simulink model "TBS_SIM"  (R2016b)
settings: Solver=ode5  StartTime=15  StopTime=30  FixedStep=0.002  RelTol=1e-3
PreLoadFcn:
  | TBS_Cai_simu_init_20170316
InitFcn:
  | TBS_Cai_simu_init_20170214
StopFcn:
  | TBS_SIMULATION_LOG
undefined symbols (not defined in the file): air_density, L1X, L2X, L3X, L3Y, MAC1, MAC2, MAC3, magnitude, motor_m0, motor_t0, ORIGIN_CD, ORIGIN_CL, ORIGIN_CM, S_seg1, S_seg2, S_seg3, y_ac
libraries: aerolibconvert2 x20, simulink x13, aerolibtransform2 x4, aerolibwind2 x3, aerolib6dof2 x1, aerolibasang x1
(part 2 of 2)

== system TBS_SIM/Variant Control System/PIDcruise/Subsystem ==
  Euler : Inport
  Constant : Constant  Value=0
  Constant1 : Constant  Value=8
  Constant2 : Constant  Value=0
  Demux : Demux  Outputs=3
  Mux : Mux  Inputs=3
  PID Controller : simulink/Continuous/PID Controller  Controller=PID  TimeDomain=Continuous-time  SampleTime=-1  IntegratorMethod=Forward Euler  FilterMethod=Forward Euler  Form=Parallel  UseFilter=on  ControllerParametersSource=internal  P=0.5  I=0.1  D=0.01  N=100  InitialConditionSource=internal  InitialConditionForIntegrator=0  InitialConditionForFilter=0  ExternalReset=none  LimitOutput=off  UpperSaturationLimit=inf  LowerSaturationLimit=-inf  LinearizeAsGain=on  AntiWindupMode=none  Kb=1  TrackingMode=off  Kt=1  PParamMin=[]  PParamMax=[]  IParamMin=[]  IParamMax=[]  DParamMin=[]  DParamMax=[]  NParamMin=[]  NParamMax=[]  KbParamMin=[]  KbParamMax=[]  KtParamMin=[]  KtParamMax=[]  POutMin=[]  POutMax=[]  IOutMin=[]  IOutMax=[]  DOutMin=[]  DOutMax=[]  NOutMin=[]  NOutMax=[]  KbOutMin=[]  KbOutMax=[]  KtOutMin=[]  KtOutMax=[]  IntegratorOutMin=[]  IntegratorOutMax=[]  FilterOutMin=[]  FilterOutMax=[]  SumOutMin=[]  SumOutMax=[]  SumI1OutMin=[]  SumI1OutMax=[]  SumI2OutMin=[]  SumI2OutMax=[]  SumI3OutMin=[]  SumI3OutMax=[]  SumDOutMin=[]  SumDOutMax=[]  SaturationOutMin=[]  SaturationOutMax=[]  IntegratorContinuousStateAttributes=''  IntegratorStateMustResolveToSignalObject=off  IntegratorRTWStateStorageClass=Auto  FilterContinuousStateAttributes=''  FilterStateMustResolveToSignalObject=off  FilterRTWStateStorageClass=Auto  DifferentiatorICPrevScaledInput=0  DifferentiatorOutMin=[]  DifferentiatorOutMax=[]
  PID Controller1 : simulink/Continuous/PID Controller  Controller=PID  TimeDomain=Continuous-time  SampleTime=-1  IntegratorMethod=Forward Euler  FilterMethod=Forward Euler  Form=Parallel  UseFilter=on  ControllerParametersSource=internal  P=0.8  I=0.5  D=0.005  N=100  InitialConditionSource=internal  InitialConditionForIntegrator=0  InitialConditionForFilter=0  ExternalReset=none  LimitOutput=off  UpperSaturationLimit=inf  LowerSaturationLimit=-inf  LinearizeAsGain=on  AntiWindupMode=none  Kb=1  TrackingMode=off  Kt=1  PParamMin=[]  PParamMax=[]  IParamMin=[]  IParamMax=[]  DParamMin=[]  DParamMax=[]  NParamMin=[]  NParamMax=[]  KbParamMin=[]  KbParamMax=[]  KtParamMin=[]  KtParamMax=[]  POutMin=[]  POutMax=[]  IOutMin=[]  IOutMax=[]  DOutMin=[]  DOutMax=[]  NOutMin=[]  NOutMax=[]  KbOutMin=[]  KbOutMax=[]  KtOutMin=[]  KtOutMax=[]  IntegratorOutMin=[]  IntegratorOutMax=[]  FilterOutMin=[]  FilterOutMax=[]  SumOutMin=[]  SumOutMax=[]  SumI1OutMin=[]  SumI1OutMax=[]  SumI2OutMin=[]  SumI2OutMax=[]  SumI3OutMin=[]  SumI3OutMax=[]  SumDOutMin=[]  SumDOutMax=[]  SaturationOutMin=[]  SaturationOutMax=[]  IntegratorContinuousStateAttributes=''  IntegratorStateMustResolveToSignalObject=off  IntegratorRTWStateStorageClass=Auto  FilterContinuousStateAttributes=''  FilterStateMustResolveToSignalObject=off  FilterRTWStateStorageClass=Auto  DifferentiatorICPrevScaledInput=0  DifferentiatorOutMin=[]  DifferentiatorOutMax=[]
  PID Controller2 : simulink/Continuous/PID Controller  Controller=PID  TimeDomain=Continuous-time  SampleTime=-1  IntegratorMethod=Forward Euler  FilterMethod=Forward Euler  Form=Parallel  UseFilter=on  ControllerParametersSource=internal  P=3  I=1.5  D=0.5  N=100  InitialConditionSource=internal  InitialConditionForIntegrator=0  InitialConditionForFilter=0  ExternalReset=none  LimitOutput=off  UpperSaturationLimit=inf  LowerSaturationLimit=-inf  LinearizeAsGain=on  AntiWindupMode=none  Kb=1  TrackingMode=off  Kt=1  PParamMin=[]  PParamMax=[]  IParamMin=[]  IParamMax=[]  DParamMin=[]  DParamMax=[]  NParamMin=[]  NParamMax=[]  KbParamMin=[]  KbParamMax=[]  KtParamMin=[]  KtParamMax=[]  POutMin=[]  POutMax=[]  IOutMin=[]  IOutMax=[]  DOutMin=[]  DOutMax=[]  NOutMin=[]  NOutMax=[]  KbOutMin=[]  KbOutMax=[]  KtOutMin=[]  KtOutMax=[]  IntegratorOutMin=[]  IntegratorOutMax=[]  FilterOutMin=[]  FilterOutMax=[]  SumOutMin=[]  SumOutMax=[]  SumI1OutMin=[]  SumI1OutMax=[]  SumI2OutMin=[]  SumI2OutMax=[]  SumI3OutMin=[]  SumI3OutMax=[]  SumDOutMin=[]  SumDOutMax=[]  SaturationOutMin=[]  SaturationOutMax=[]  IntegratorContinuousStateAttributes=''  IntegratorStateMustResolveToSignalObject=off  IntegratorRTWStateStorageClass=Auto  FilterContinuousStateAttributes=''  FilterStateMustResolveToSignalObject=off  FilterRTWStateStorageClass=Auto  DifferentiatorICPrevScaledInput=0  DifferentiatorOutMin=[]  DifferentiatorOutMax=[]
  Sum : Sum  Inputs=+-|
  Sum1 : Sum  Inputs=+-|
  Sum2 : Sum  Inputs=+-|
  Out1 : Outport
  wires:
  Euler/1 -> Demux/1
  Sum/1 -> PID Controller/1
  Demux/1 -> Sum/2
  Constant/1 -> Sum/1
  Sum1/1 -> PID Controller1/1
  Demux/2 -> Sum1/2
  Constant1/1 -> Sum1/1
  Sum2/1 -> PID Controller2/1
  Demux/3 -> Sum2/2
  Constant2/1 -> Sum2/1
  PID Controller/1 -> Mux/1
  PID Controller1/1 -> Mux/2
  PID Controller2/1 -> Mux/3
  Mux/1 -> Out1/1

== system TBS_SIM/Variant Control System/PIDcruise/Subsystem1 ==
  Velocity : Inport
  Constant : Constant  Value=10
  PID Controller2 : simulink/Continuous/PID Controller  Controller=PID  TimeDomain=Continuous-time  SampleTime=-1  IntegratorMethod=Forward Euler  FilterMethod=Forward Euler  Form=Parallel  UseFilter=on  ControllerParametersSource=internal  P=3  I=1  D=0.5  N=100  InitialConditionSource=internal  InitialConditionForIntegrator=0  InitialConditionForFilter=0  ExternalReset=none  LimitOutput=off  UpperSaturationLimit=inf  LowerSaturationLimit=-inf  LinearizeAsGain=on  AntiWindupMode=none  Kb=1  TrackingMode=off  Kt=1  PParamMin=[]  PParamMax=[]  IParamMin=[]  IParamMax=[]  DParamMin=[]  DParamMax=[]  NParamMin=[]  NParamMax=[]  KbParamMin=[]  KbParamMax=[]  KtParamMin=[]  KtParamMax=[]  POutMin=[]  POutMax=[]  IOutMin=[]  IOutMax=[]  DOutMin=[]  DOutMax=[]  NOutMin=[]  NOutMax=[]  KbOutMin=[]  KbOutMax=[]  KtOutMin=[]  KtOutMax=[]  IntegratorOutMin=[]  IntegratorOutMax=[]  FilterOutMin=[]  FilterOutMax=[]  SumOutMin=[]  SumOutMax=[]  SumI1OutMin=[]  SumI1OutMax=[]  SumI2OutMin=[]  SumI2OutMax=[]  SumI3OutMin=[]  SumI3OutMax=[]  SumDOutMin=[]  SumDOutMax=[]  SaturationOutMin=[]  SaturationOutMax=[]  IntegratorContinuousStateAttributes=''  IntegratorStateMustResolveToSignalObject=off  IntegratorRTWStateStorageClass=Auto  FilterContinuousStateAttributes=''  FilterStateMustResolveToSignalObject=off  FilterRTWStateStorageClass=Auto  DifferentiatorICPrevScaledInput=0  DifferentiatorOutMin=[]  DifferentiatorOutMax=[]
  Selector : Selector  InputPortWidth=3  IndexOptions=Index vector (dialog)  Indices=[1]  OutputSizes=1
  Sum2 : Sum  Inputs=+-|
  Out1 : Outport
  wires:
  Velocity/1 -> Selector/1
  Sum2/1 -> PID Controller2/1
  PID Controller2/1 -> Out1/1
  Selector/1 -> Sum2/2
  Constant/1 -> Sum2/1

== system TBS_SIM/Variant Control System/PIDcruise/Subsystem2 ==
  Moment : Inport
  Fprce : Inport  Port=2
  Demux : Demux  Outputs=3
  Gain : Gain  Gain=2000
  Gain1 : Gain  Gain=-50
  Gain2 : Gain  Gain=50
  Gain3 : Gain  Gain=-1000
  Mux : Mux
  Sum : Sum  Inputs=++|
  Sum1 : Sum  Inputs=-+|
  Sum2 : Sum  Inputs=2
  Sum3 : Sum  Inputs=-+
  Out1 : Outport
  wires:
  Fprce/1 -> Gain/1
  Moment/1 -> Demux/1
  Demux/2 -> Gain1/1
  Demux/1 -> Gain2/1
  Demux/3 -> Gain3/1
  Gain3/1 -> Sum/1, Sum1/1
  Gain/1 -> Sum1/2, Sum/2
  Sum/1 -> Mux/1
  Sum1/1 -> Mux/2
  Gain2/1 -> Sum3/1, Sum2/1
  Gain1/1 -> Sum3/2, Sum2/2
  Sum2/1 -> Mux/4
  Sum3/1 -> Mux/3
  Mux/1 -> Out1/1

== system TBS_SIM/Variant Control System/Transition/Trans ==
  State : Inport
  Bus Selector : BusSelector  OutputSignals=v_b,euler
  Chart : Stateflow chart  TreatAsAtomicUnit=on
  Cruise Controller : Subsystem
  Demux : Demux  Outputs=3
  Demux1 : Demux  Outputs=3
  Scope : Scope
  Switch : Switch  Criteria=u2 ~= 0
  Terminator{,1..3} (4 alike) : Terminator
  Transition Controller : Subsystem
  Commands : Outport
  wires:
  Demux1/3 -> Terminator3/1
  Demux1/1 -> Terminator2/1
  Demux/3 -> Terminator1/1
  Demux/2 -> Terminator/1
  Demux1/2 -> Chart/2(pitch)
  Bus Selector/2 -> Demux1/1  "<euler>"
  Demux/1 -> Chart/1(v)
  Bus Selector/1 -> Demux/1  "<v_b>"
  Switch/1 -> Commands/1
  State/1 -> Transition Controller/1(state 1), Bus Selector/1, Cruise Controller/1(State)
  Cruise Controller/1("Commands ") -> Switch/3
  Transition Controller/1("Command ") -> Switch/1
  Chart/1(trans_mode) -> Switch/2, Scope/1

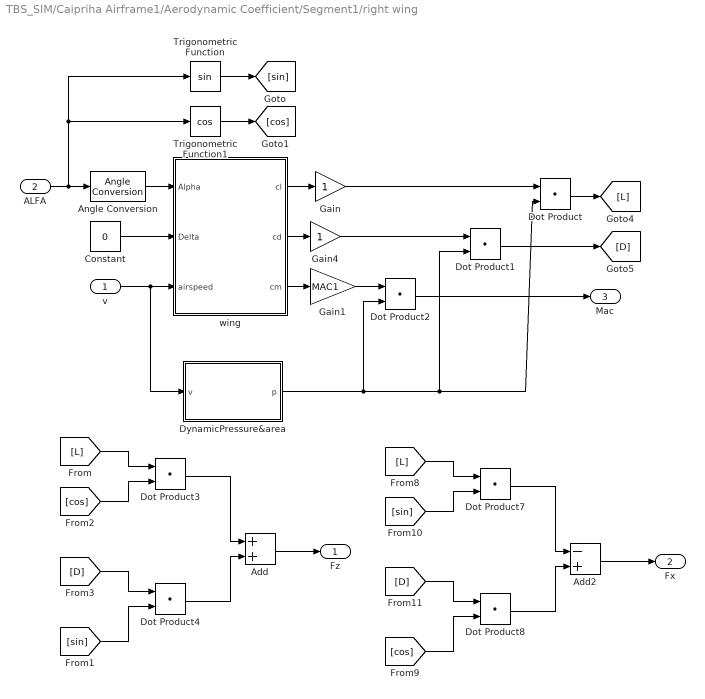
== system TBS_SIM/Caipriha Airframe1/Aerodynamic Coefficient/Segment1/right wing ==
  v : Inport
  "ALFA " : Inport  Port=2
  Add : Sum
  Add2 : Sum  Inputs=-+
  Angle Conversion : aerolibconvert2/Angle Conversion  IU=rad  OU=deg
  Constant : Constant  Value=0
  Dot Product{,1..4,7..8} (7 alike) : DotProduct  InputSameDT=on  OutDataTypeStr=Inherit: Inherit via internal rule
  DynamicPressure&area : Subsystem
  Gain : Gain
  Gain1 : Gain  Gain=MAC1
  Gain4 : Gain
  Trigonometric Function : Trigonometry
  Trigonometric Function1 : Trigonometry  Operator=cos
  wing : Subsystem
  Fz : Outport
  Fx : Outport  Port=2
  Mac : Outport  Port=3
  wires:
  wing/3(cm) -> Gain1/1
  Gain4/1 -> Dot Product1/1
  Gain/1 -> Dot Product/1
  wing/1(cl) -> Gain/1
  v/1 -> DynamicPressure&area/1(v), wing/3(airspeed)
  Constant/1 -> wing/2(Delta)
  DynamicPressure&area/1(p) -> Dot Product/2, Dot Product1/2, Dot Product2/2
  wing/2(cd) -> Gain4/1
  Gain1/1 -> Dot Product2/1
  Dot Product2/1 -> Mac/1
  Angle Conversion/1 -> wing/1(Alpha)
  Trigonometric Function/1 -> [sin]
  "ALFA "/1 -> Trigonometric Function/1, Trigonometric Function1/1, Angle Conversion/1
  Trigonometric Function1/1 -> [cos]
  Dot Product/1 -> [L]
  Dot Product1/1 -> [D]
  [L] -> Dot Product3/1
  [cos] -> Dot Product3/2
  [D] -> Dot Product4/1
  [sin] -> Dot Product4/2
  Dot Product3/1 -> Add/1
  Dot Product4/1 -> Add/2
  Add/1 -> Fz/1
  [L] -> Dot Product7/1
  [sin] -> Dot Product7/2
  [D] -> Dot Product8/1
  [cos] -> Dot Product8/2
  Dot Product7/1 -> Add2/1
  Dot Product8/1 -> Add2/2
  Add2/1 -> Fx/1

== system TBS_SIM/Caipriha Airframe1/Aerodynamic Coefficient/Segment2/immersed velocity ==
  alpha : Inport
  "t1 " : Inport  Port=2
  t2 : Inport  Port=3
  airspeed : Inport  Port=4
  "Immersed velocity " : Subsystem
  Immersed velocity 1 : Subsystem
  v1 : Outport
  v2 : Outport  Port=2
  wires:
  airspeed/1 -> "Immersed velocity "/2(airspeed), Immersed velocity 1/2(airspeed)
  alpha/1 -> Immersed velocity 1/3(alfa), "Immersed velocity "/3(alfa)
  Immersed velocity 1/1(v) -> v2/1
  "Immersed velocity "/1(v) -> v1/1
  t2/1 -> Immersed velocity 1/1(T)
  "t1 "/1 -> "Immersed velocity "/1(T)

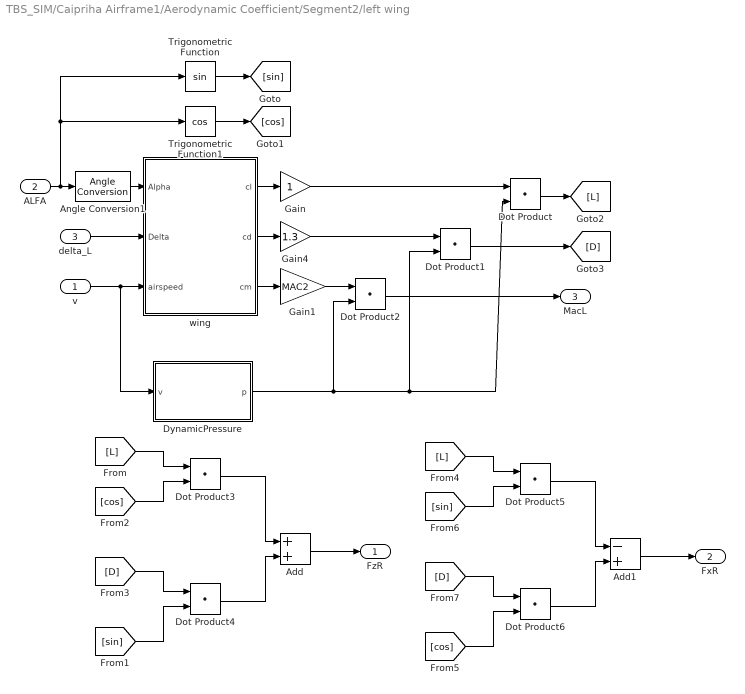
== system TBS_SIM/Caipriha Airframe1/Aerodynamic Coefficient/Segment2/left wing ==
  v : Inport
  "ALFA " : Inport  Port=2
  delta_L : Inport  Port=3
  Add : Sum
  Add1 : Sum  Inputs=-+
  Angle Conversion1 : aerolibconvert2/Angle Conversion  IU=rad  OU=deg
  Dot Product{,1..6} (7 alike) : DotProduct  InputSameDT=on  OutDataTypeStr=Inherit: Inherit via internal rule
  DynamicPressure : Subsystem
  Gain : Gain
  Gain1 : Gain  Gain=MAC2
  Gain4 : Gain  Gain=1.3
  Trigonometric Function : Trigonometry
  Trigonometric Function1 : Trigonometry  Operator=cos
  wing : Subsystem
  FzR : Outport
  FxR : Outport  Port=2
  MacL : Outport  Port=3
  wires:
  wing/3(cm) -> Gain1/1
  Gain4/1 -> Dot Product1/1
  Gain/1 -> Dot Product/1
  wing/1(cl) -> Gain/1
  v/1 -> DynamicPressure/1(v), wing/3(airspeed)
  delta_L/1 -> wing/2(Delta)
  DynamicPressure/1(p) -> Dot Product/2, Dot Product1/2, Dot Product2/2
  wing/2(cd) -> Gain4/1
  Gain1/1 -> Dot Product2/1
  Dot Product2/1 -> MacL/1
  Angle Conversion1/1 -> wing/1(Alpha)
  Trigonometric Function/1 -> [sin]
  "ALFA "/1 -> Trigonometric Function/1, Trigonometric Function1/1, Angle Conversion1/1
  Trigonometric Function1/1 -> [cos]
  Dot Product/1 -> [L]
  Dot Product1/1 -> [D]
  [L] -> Dot Product3/1
  [cos] -> Dot Product3/2
  [D] -> Dot Product4/1
  [sin] -> Dot Product4/2
  Dot Product3/1 -> Add/1
  Dot Product4/1 -> Add/2
  Add/1 -> FzR/1
  [L] -> Dot Product5/1
  [sin] -> Dot Product5/2
  [D] -> Dot Product6/1
  [cos] -> Dot Product6/2
  Dot Product5/1 -> Add1/1
  Dot Product6/1 -> Add1/2
  Add1/1 -> FxR/1

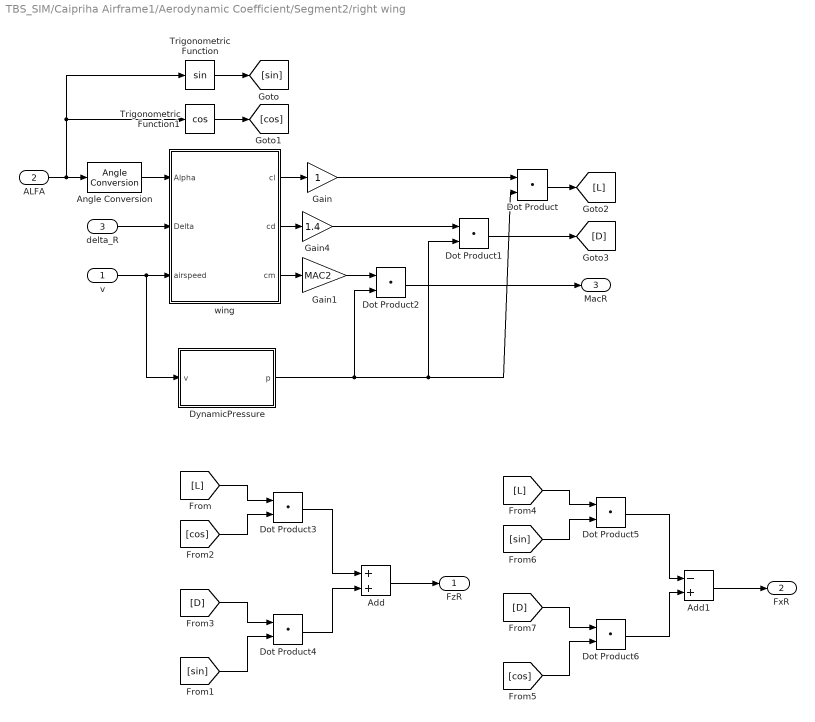
== system TBS_SIM/Caipriha Airframe1/Aerodynamic Coefficient/Segment2/right wing ==
  v : Inport
  "ALFA " : Inport  Port=2
  delta_R : Inport  Port=3
  Add : Sum
  Add1 : Sum  Inputs=-+
  Angle Conversion : aerolibconvert2/Angle Conversion  IU=rad  OU=deg
  Dot Product{,1..6} (7 alike) : DotProduct  InputSameDT=on  OutDataTypeStr=Inherit: Inherit via internal rule
  DynamicPressure : Subsystem
  Gain : Gain
  Gain1 : Gain  Gain=MAC2
  Gain4 : Gain  Gain=1.4
  Trigonometric Function : Trigonometry
  Trigonometric Function1 : Trigonometry  Operator=cos
  wing : Subsystem
  FzR : Outport
  FxR : Outport  Port=2
  MacR : Outport  Port=3
  wires:
  wing/3(cm) -> Gain1/1
  Gain4/1 -> Dot Product1/1
  Gain/1 -> Dot Product/1
  wing/1(cl) -> Gain/1
  v/1 -> DynamicPressure/1(v), wing/3(airspeed)
  delta_R/1 -> wing/2(Delta)
  DynamicPressure/1(p) -> Dot Product/2, Dot Product1/2, Dot Product2/2
  wing/2(cd) -> Gain4/1
  Gain1/1 -> Dot Product2/1
  Dot Product2/1 -> MacR/1
  Angle Conversion/1 -> wing/1(Alpha)
  Trigonometric Function/1 -> [sin]
  "ALFA "/1 -> Trigonometric Function/1, Trigonometric Function1/1, Angle Conversion/1
  Trigonometric Function1/1 -> [cos]
  Dot Product/1 -> [L]
  Dot Product1/1 -> [D]
  [L] -> Dot Product3/1
  [cos] -> Dot Product3/2
  [D] -> Dot Product4/1
  [sin] -> Dot Product4/2
  Dot Product3/1 -> Add/1
  Dot Product4/1 -> Add/2
  Add/1 -> FzR/1
  [L] -> Dot Product5/1
  [sin] -> Dot Product5/2
  [D] -> Dot Product6/1
  [cos] -> Dot Product6/2
  Dot Product5/1 -> Add1/1
  Dot Product6/1 -> Add1/2
  Add1/1 -> FxR/1

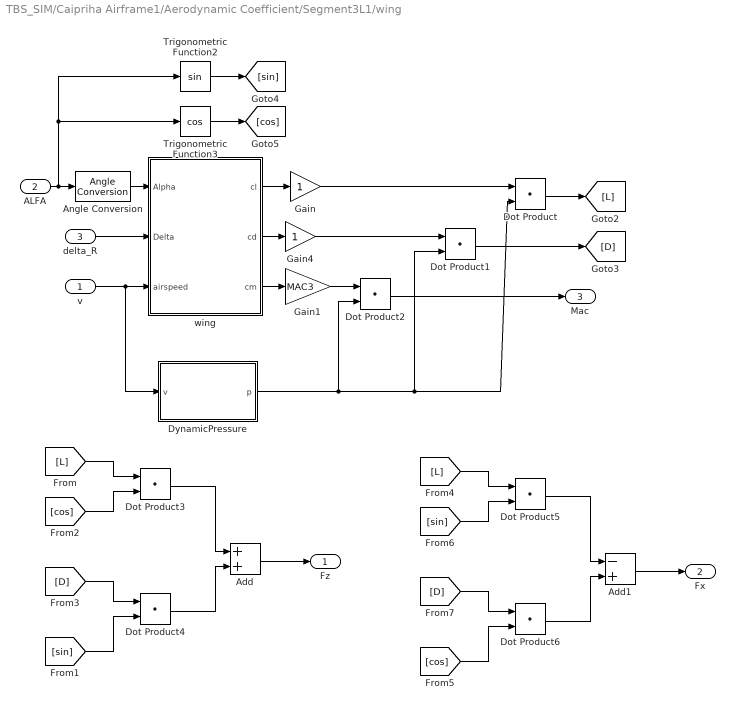
== system TBS_SIM/Caipriha Airframe1/Aerodynamic Coefficient/Segment3L1/wing ==
  v : Inport
  "ALFA " : Inport  Port=2
  delta_R : Inport  Port=3
  Add : Sum
  Add1 : Sum  Inputs=-+
  Angle Conversion : aerolibconvert2/Angle Conversion  IU=rad  OU=deg
  Dot Product{,1..6} (7 alike) : DotProduct  InputSameDT=on  OutDataTypeStr=Inherit: Inherit via internal rule
  DynamicPressure : Subsystem
  Gain : Gain
  Gain1 : Gain  Gain=MAC3
  Gain4 : Gain
  Trigonometric Function2 : Trigonometry
  Trigonometric Function3 : Trigonometry  Operator=cos
  wing : Subsystem
  Fz : Outport
  Fx : Outport  Port=2
  Mac : Outport  Port=3
  wires:
  wing/3(cm) -> Gain1/1
  Gain4/1 -> Dot Product1/1
  Gain/1 -> Dot Product/1
  wing/1(cl) -> Gain/1
  v/1 -> DynamicPressure/1(v), wing/3(airspeed)
  delta_R/1 -> wing/2(Delta)
  DynamicPressure/1(p) -> Dot Product/2, Dot Product1/2, Dot Product2/2
  wing/2(cd) -> Gain4/1
  Gain1/1 -> Dot Product2/1
  Dot Product2/1 -> Mac/1
  Angle Conversion/1 -> wing/1(Alpha)
  Trigonometric Function2/1 -> [sin]
  "ALFA "/1 -> Trigonometric Function2/1, Trigonometric Function3/1, Angle Conversion/1
  Trigonometric Function3/1 -> [cos]
  Dot Product/1 -> [L]
  Dot Product1/1 -> [D]
  [L] -> Dot Product3/1
  [cos] -> Dot Product3/2
  [D] -> Dot Product4/1
  [sin] -> Dot Product4/2
  Dot Product3/1 -> Add/1
  Dot Product4/1 -> Add/2
  Add/1 -> Fz/1
  [L] -> Dot Product5/1
  [sin] -> Dot Product5/2
  [D] -> Dot Product6/1
  [cos] -> Dot Product6/2
  Dot Product5/1 -> Add1/1
  Dot Product6/1 -> Add1/2
  Add1/1 -> Fx/1

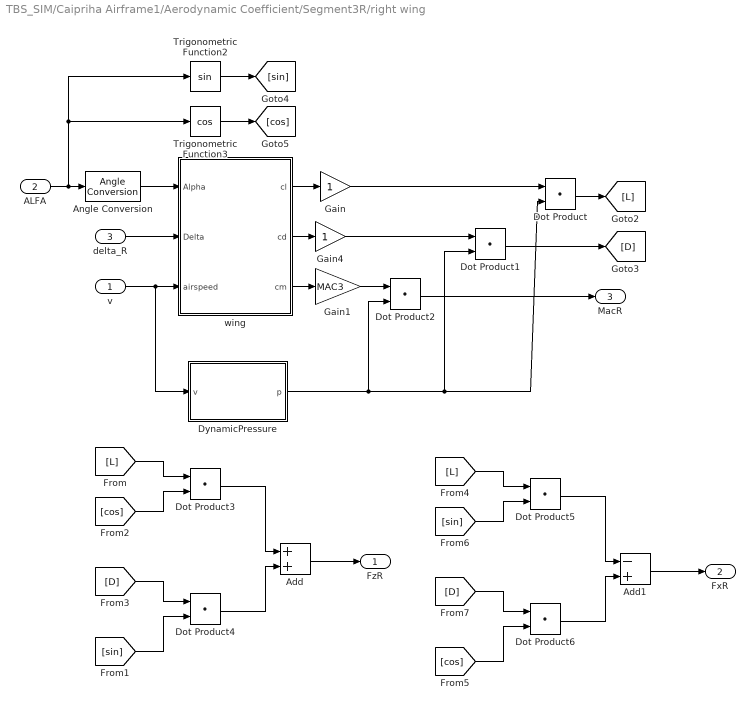
== system TBS_SIM/Caipriha Airframe1/Aerodynamic Coefficient/Segment3R/right wing ==
  v : Inport
  "ALFA " : Inport  Port=2
  delta_R : Inport  Port=3
  Add : Sum
  Add1 : Sum  Inputs=-+
  Angle Conversion : aerolibconvert2/Angle Conversion  IU=rad  OU=deg
  Dot Product{,1..6} (7 alike) : DotProduct  InputSameDT=on  OutDataTypeStr=Inherit: Inherit via internal rule
  DynamicPressure : Subsystem
  Gain : Gain
  Gain1 : Gain  Gain=MAC3
  Gain4 : Gain
  Trigonometric Function2 : Trigonometry
  Trigonometric Function3 : Trigonometry  Operator=cos
  wing : Subsystem
  FzR : Outport
  FxR : Outport  Port=2
  MacR : Outport  Port=3
  wires:
  wing/3(cm) -> Gain1/1
  Gain4/1 -> Dot Product1/1
  Gain/1 -> Dot Product/1
  wing/1(cl) -> Gain/1
  v/1 -> DynamicPressure/1(v), wing/3(airspeed)
  delta_R/1 -> wing/2(Delta)
  DynamicPressure/1(p) -> Dot Product/2, Dot Product1/2, Dot Product2/2
  wing/2(cd) -> Gain4/1
  Gain1/1 -> Dot Product2/1
  Dot Product2/1 -> MacR/1
  Angle Conversion/1 -> wing/1(Alpha)
  Trigonometric Function2/1 -> [sin]
  "ALFA "/1 -> Trigonometric Function2/1, Trigonometric Function3/1, Angle Conversion/1
  Trigonometric Function3/1 -> [cos]
  Dot Product/1 -> [L]
  Dot Product1/1 -> [D]
  [L] -> Dot Product3/1
  [cos] -> Dot Product3/2
  [D] -> Dot Product4/1
  [sin] -> Dot Product4/2
  Dot Product3/1 -> Add/1
  Dot Product4/1 -> Add/2
  Add/1 -> FzR/1
  [L] -> Dot Product5/1
  [sin] -> Dot Product5/2
  [D] -> Dot Product6/1
  [cos] -> Dot Product6/2
  Dot Product5/1 -> Add1/1
  Dot Product6/1 -> Add1/2
  Add1/1 -> FxR/1

== system TBS_SIM/Variant Control System/Transition/Trans/Cruise Controller ==
  State : Inport
  Bus Selector : BusSelector  OutputSignals=v_e,x_e,DCM,omega,v_b,euler
  Cruise : Subsystem  VariantControl=CruseController
  Mux1 : Mux  Inputs=2
  "Commands " : Outport
  wires:
  Mux1/1 -> "Commands "/1
  Bus Selector/6 -> Cruise/6(Euler)  "<euler>"
  State/1 -> Bus Selector/1
  Cruise/1(RS) -> Mux1/1
  Cruise/2("Actuator ") -> Mux1/2
  Bus Selector/5 -> Cruise/5(V_b)  "<v_b>"
  Bus Selector/4 -> Cruise/4(pqr)  "<omega>"
  Bus Selector/3 -> Cruise/3(DCM)  "<DCM>"
  Bus Selector/2 -> Cruise/2(Xe)  "<x_e>"
  Bus Selector/1 -> Cruise/1(Ve)  "<v_e>"

== system TBS_SIM/Variant Control System/Transition/Trans/Transition Controller ==
  state 1 : Inport
  Bus Selector1 : BusSelector  OutputSignals=v_e,x_e,DCM,omega
  Constant : Constant  Value=[0,0,0]
  Constant2 : Constant  Value=0
  Hover : Subsystem  VariantControl=HoveringController
  Mux : Mux  Inputs=3
  Mux2 : Mux  Inputs=2
  Ramp : simulink/Sources/Ramp  slope=0.8  start=1  X0=0
  Saturation4 : Saturate  UpperLimit=3.5  LowerLimit=0
  "Command " : Outport
  wires:
  Mux2/1 -> "Command "/1
  Hover/2("Actuator ") -> Mux2/2
  Hover/1(RS) -> Mux2/1
  state 1/1 -> Bus Selector1/1
  Bus Selector1/1 -> Hover/1(Ve)  "<v_e>"
  Bus Selector1/2 -> Hover/2(Xe)  "<x_e>"
  Bus Selector1/3 -> Hover/3(DCM)  "<DCM>"
  Bus Selector1/4 -> Hover/4(pqr)  "<omega>"
  Constant/1 -> Hover/6(des_p)
  Mux/1 -> Hover/5(des_v)
  Constant2/1 -> Mux/1, Mux/2
  Saturation4/1 -> Mux/3
  Ramp/1 -> Saturation4/1

== system TBS_SIM/Caipriha Airframe1/Aerodynamic Coefficient/Segment1/right wing/DynamicPressure&area ==
  v : Inport
  Gain1 : Gain  Gain=air_density
  Gain2 : Gain  Gain=0.5
  Gain3 : Gain  Gain=S_seg1*2
  Math Function : Math  Operator=magnitude^2  SaturateOnIntegerOverflow=on
  p : Outport
  wires:
  Gain3/1 -> p/1
  Gain2/1 -> Gain3/1
  Gain1/1 -> Gain2/1
  Math Function/1 -> Gain1/1
  v/1 -> Math Function/1

== system TBS_SIM/Caipriha Airframe1/Aerodynamic Coefficient/Segment1/right wing/wing ==
  Alpha : Inport
  Delta : Inport  Port=2
  airspeed : Inport  Port=3
  AirspeedLookup : PreLookup  BreakpointsData=as  BeginIndexSearchUsingPreviousIndexResult=on  ExtrapMethod=Linear
  AlphaLookup : PreLookup  BreakpointsData=alpha_vec_0  BeginIndexSearchUsingPreviousIndexResult=on  ExtrapMethod=Linear
  CD : Interpolation_n-D  NumberOfTableDimensions=3  Table=ORIGIN_CD  ExtrapMethod=Clip  DiagnosticForOutOfRangeInput=Warning  InternalRulePriority=Speed
      settings: InputPortMap=u0,u1,u2,u3,u4,u5
  CD1 : Interpolation_n-D  NumberOfTableDimensions=3  Table=ORIGIN_CM  ExtrapMethod=Clip  DiagnosticForOutOfRangeInput=Warning  InternalRulePriority=Speed
      settings: InputPortMap=u0,u1,u2,u3,u4,u5
  CL : Interpolation_n-D  NumberOfTableDimensions=3  Table=ORIGIN_CL  ExtrapMethod=Clip  DiagnosticForOutOfRangeInput=Warning  InternalRulePriority=Speed
      settings: InputPortMap=u0,u1,u2,u3,u4,u5
  DeltaLookup : PreLookup  BreakpointsData=ORIGIN_DELTA  BeginIndexSearchUsingPreviousIndexResult=on  ExtrapMethod=Linear
  cl : Outport
  cd : Outport  Port=2
  cm : Outport  Port=3
  wires:
  Alpha/1 -> AlphaLookup/1
  airspeed/1 -> AirspeedLookup/1
  DeltaLookup/1 -> CD1/5, CL/5, CD/5
  DeltaLookup/2 -> CD1/6, CL/6, CD/6
  CL/1 -> cl/1
  AirspeedLookup/1 -> CD1/1, CD/1, CL/1
  AirspeedLookup/2 -> CD1/2, CD/2, CL/2
  AlphaLookup/1 -> CD/3, CD1/3, CL/3
  AlphaLookup/2 -> CD1/4, CD/4, CL/4
  CD/1 -> cd/1
  CD1/1 -> cm/1
  Delta/1 -> DeltaLookup/1

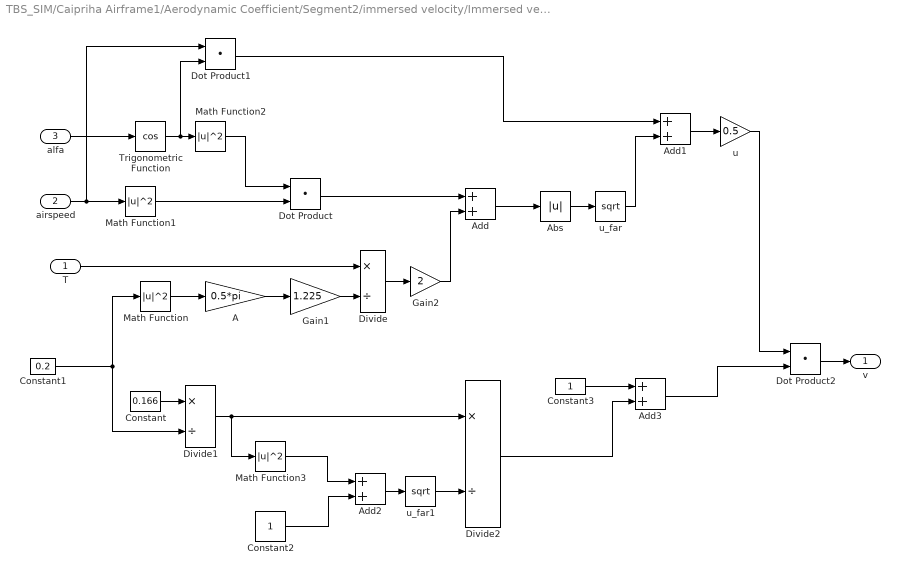
== system TBS_SIM/Caipriha Airframe1/Aerodynamic Coefficient/Segment2/immersed velocity/Immersed velocity  ==
  T : Inport
  airspeed : Inport  Port=2
  alfa : Inport  Port=3
  A : Gain  Gain=0.5*pi
  Abs : Abs
  Add{,1..3} (4 alike) : Sum
  Constant : Constant  Value=0.166
  Constant1 : Constant  Value=0.2
  Constant2 : Constant
  Constant3 : Constant
  Divide : Product  Inputs=*/
  Divide1 : Product  Inputs=*/
  Divide2 : Product  Inputs=*/
  Dot Product : DotProduct  InputSameDT=on  OutDataTypeStr=Inherit: Inherit via internal rule
  Dot Product1 : DotProduct  InputSameDT=on  OutDataTypeStr=Inherit: Inherit via internal rule
  Dot Product2 : DotProduct  InputSameDT=on  OutDataTypeStr=Inherit: Inherit via internal rule
  Gain1 : Gain  Gain=1.225
  Gain2 : Gain  Gain=2
  Math Function{,1..3} (4 alike) : Math  Operator=magnitude^2  SaturateOnIntegerOverflow=on
  Trigonometric Function : Trigonometry  Operator=cos
  u : Gain  Gain=0.5
  u_far : Sqrt  SaturateOnIntegerOverflow=on
  u_far1 : Sqrt  SaturateOnIntegerOverflow=on
  v : Outport
  wires:
  Add3/1 -> Dot Product2/2
  Divide2/1 -> Add3/2
  u/1 -> Dot Product2/1
  Constant3/1 -> Add3/1
  Divide1/1 -> Divide2/1, Math Function3/1
  u_far1/1 -> Divide2/2
  Add2/1 -> u_far1/1
  Constant2/1 -> Add2/2
  Math Function3/1 -> Add2/1
  Constant/1 -> Divide1/1
  Add1/1 -> u/1
  Dot Product1/1 -> Add1/1
  u_far/1 -> Add1/2
  Math Function2/1 -> Dot Product/1
  Trigonometric Function/1 -> Math Function2/1, Dot Product1/2
  Abs/1 -> u_far/1
  Add/1 -> Abs/1
  Gain2/1 -> Add/2
  Dot Product/1 -> Add/1
  Math Function1/1 -> Dot Product/2
  alfa/1 -> Trigonometric Function/1
  airspeed/1 -> Math Function1/1, Dot Product1/1
  Divide/1 -> Gain2/1
  T/1 -> Divide/1
  Gain1/1 -> Divide/2
  A/1 -> Gain1/1
  Math Function/1 -> A/1
  Constant1/1 -> Math Function/1, Divide1/2
  Dot Product2/1 -> v/1

== system TBS_SIM/Caipriha Airframe1/Aerodynamic Coefficient/Segment2/immersed velocity/Immersed velocity 1 ==
  T : Inport
  airspeed : Inport  Port=2
  alfa : Inport  Port=3
  A : Gain  Gain=0.5*pi
  Abs : Abs
  Add{,1..3} (4 alike) : Sum
  Constant : Constant  Value=0.166
  Constant1 : Constant  Value=0.2
  Constant2 : Constant
  Constant3 : Constant
  Divide : Product  Inputs=*/
  Divide1 : Product  Inputs=*/
  Divide2 : Product  Inputs=*/
  Dot Product : DotProduct  InputSameDT=on  OutDataTypeStr=Inherit: Inherit via internal rule
  Dot Product1 : DotProduct  InputSameDT=on  OutDataTypeStr=Inherit: Inherit via internal rule
  Dot Product2 : DotProduct  InputSameDT=on  OutDataTypeStr=Inherit: Inherit via internal rule
  Gain1 : Gain  Gain=1.225
  Gain2 : Gain  Gain=2
  Math Function{,1..3} (4 alike) : Math  Operator=magnitude^2  SaturateOnIntegerOverflow=on
  Trigonometric Function : Trigonometry  Operator=cos
  u : Gain  Gain=0.5
  u_far : Sqrt  SaturateOnIntegerOverflow=on
  u_far1 : Sqrt  SaturateOnIntegerOverflow=on
  v : Outport
  wires:
  Add3/1 -> Dot Product2/2
  Divide2/1 -> Add3/2
  Constant3/1 -> Add3/1
  Dot Product2/1 -> v/1
  u/1 -> Dot Product2/1
  Divide1/1 -> Math Function3/1, Divide2/1
  u_far1/1 -> Divide2/2
  Add2/1 -> u_far1/1
  Constant2/1 -> Add2/2
  Math Function3/1 -> Add2/1
  Constant/1 -> Divide1/1
  Add1/1 -> u/1
  Dot Product1/1 -> Add1/1
  u_far/1 -> Add1/2
  Math Function2/1 -> Dot Product/1
  Trigonometric Function/1 -> Math Function2/1, Dot Product1/2
  Abs/1 -> u_far/1
  Add/1 -> Abs/1
  Gain2/1 -> Add/2
  Dot Product/1 -> Add/1
  Math Function1/1 -> Dot Product/2
  alfa/1 -> Trigonometric Function/1
  airspeed/1 -> Math Function1/1, Dot Product1/1
  Divide/1 -> Gain2/1
  T/1 -> Divide/1
  Gain1/1 -> Divide/2
  A/1 -> Gain1/1
  Math Function/1 -> A/1
  Constant1/1 -> Math Function/1, Divide1/2

== system TBS_SIM/Caipriha Airframe1/Aerodynamic Coefficient/Segment2/left wing/DynamicPressure ==
  v : Inport
  Gain1 : Gain  Gain=air_density
  Gain2 : Gain  Gain=0.5
  Gain3 : Gain  Gain=S_seg2
  Math Function : Math  Operator=magnitude^2  SaturateOnIntegerOverflow=on
  p : Outport
  wires:
  Gain3/1 -> p/1
  Gain2/1 -> Gain3/1
  Gain1/1 -> Gain2/1
  Math Function/1 -> Gain1/1
  v/1 -> Math Function/1

== system TBS_SIM/Caipriha Airframe1/Aerodynamic Coefficient/Segment2/left wing/wing ==
  Alpha : Inport
  Delta : Inport  Port=2
  airspeed : Inport  Port=3
  AirspeedLookup : PreLookup  BreakpointsData=as  BeginIndexSearchUsingPreviousIndexResult=on  ExtrapMethod=Linear
  AlphaLookup : PreLookup  BreakpointsData=alpha_vec_0  BeginIndexSearchUsingPreviousIndexResult=on  ExtrapMethod=Linear
  CD : Interpolation_n-D  NumberOfTableDimensions=3  Table=ORIGIN_CD  ExtrapMethod=Clip  DiagnosticForOutOfRangeInput=Warning  InternalRulePriority=Speed
      settings: InputPortMap=u0,u1,u2,u3,u4,u5
  CD1 : Interpolation_n-D  NumberOfTableDimensions=3  Table=ORIGIN_CM  ExtrapMethod=Clip  DiagnosticForOutOfRangeInput=Warning  InternalRulePriority=Speed
      settings: InputPortMap=u0,u1,u2,u3,u4,u5
  CL : Interpolation_n-D  NumberOfTableDimensions=3  Table=ORIGIN_CL  ExtrapMethod=Clip  DiagnosticForOutOfRangeInput=Warning  InternalRulePriority=Speed
      settings: InputPortMap=u0,u1,u2,u3,u4,u5
  DeltaLookup : PreLookup  BreakpointsData=ORIGIN_DELTA  BeginIndexSearchUsingPreviousIndexResult=on  ExtrapMethod=Linear
  cl : Outport
  cd : Outport  Port=2
  cm : Outport  Port=3
  wires:
  Alpha/1 -> AlphaLookup/1
  airspeed/1 -> AirspeedLookup/1
  DeltaLookup/1 -> CD1/5, CL/5, CD/5
  DeltaLookup/2 -> CD1/6, CL/6, CD/6
  CL/1 -> cl/1
  AirspeedLookup/1 -> CD1/1, CD/1, CL/1
  AirspeedLookup/2 -> CD1/2, CD/2, CL/2
  AlphaLookup/1 -> CD/3, CD1/3, CL/3
  AlphaLookup/2 -> CD1/4, CD/4, CL/4
  CD/1 -> cd/1
  CD1/1 -> cm/1
  Delta/1 -> DeltaLookup/1

== system TBS_SIM/Caipriha Airframe1/Aerodynamic Coefficient/Segment2/right wing/DynamicPressure ==
  v : Inport
  Gain1 : Gain  Gain=air_density
  Gain2 : Gain  Gain=0.5
  Gain3 : Gain  Gain=S_seg2
  Math Function : Math  Operator=magnitude^2  SaturateOnIntegerOverflow=on
  p : Outport
  wires:
  Gain3/1 -> p/1
  Gain2/1 -> Gain3/1
  Gain1/1 -> Gain2/1
  Math Function/1 -> Gain1/1
  v/1 -> Math Function/1

== system TBS_SIM/Caipriha Airframe1/Aerodynamic Coefficient/Segment2/right wing/wing ==
  Alpha : Inport
  Delta : Inport  Port=2
  airspeed : Inport  Port=3
  AirspeedLookup : PreLookup  BreakpointsData=as  BeginIndexSearchUsingPreviousIndexResult=on  ExtrapMethod=Linear
  AlphaLookup : PreLookup  BreakpointsData=alpha_vec_0  BeginIndexSearchUsingPreviousIndexResult=on  ExtrapMethod=Linear
  CD : Interpolation_n-D  NumberOfTableDimensions=3  Table=ORIGIN_CD  ExtrapMethod=Clip  DiagnosticForOutOfRangeInput=Warning  InternalRulePriority=Speed
      settings: InputPortMap=u0,u1,u2,u3,u4,u5
  CD1 : Interpolation_n-D  NumberOfTableDimensions=3  Table=ORIGIN_CM  ExtrapMethod=Clip  DiagnosticForOutOfRangeInput=Warning  InternalRulePriority=Speed
      settings: InputPortMap=u0,u1,u2,u3,u4,u5
  CL : Interpolation_n-D  NumberOfTableDimensions=3  Table=ORIGIN_CL  ExtrapMethod=Clip  DiagnosticForOutOfRangeInput=Warning  InternalRulePriority=Speed
      settings: InputPortMap=u0,u1,u2,u3,u4,u5
  DeltaLookup : PreLookup  BreakpointsData=ORIGIN_DELTA  BeginIndexSearchUsingPreviousIndexResult=on  ExtrapMethod=Linear
  cl : Outport
  cd : Outport  Port=2
  cm : Outport  Port=3
  wires:
  Alpha/1 -> AlphaLookup/1
  airspeed/1 -> AirspeedLookup/1
  DeltaLookup/1 -> CD1/5, CL/5, CD/5
  DeltaLookup/2 -> CD1/6, CL/6, CD/6
  CL/1 -> cl/1
  AirspeedLookup/1 -> CD1/1, CD/1, CL/1
  AirspeedLookup/2 -> CD1/2, CD/2, CL/2
  AlphaLookup/1 -> CD/3, CD1/3, CL/3
  AlphaLookup/2 -> CD1/4, CD/4, CL/4
  CD/1 -> cd/1
  CD1/1 -> cm/1
  Delta/1 -> DeltaLookup/1

== system TBS_SIM/Caipriha Airframe1/Aerodynamic Coefficient/Segment3L1/wing/DynamicPressure ==
  v : Inport
  Gain1 : Gain  Gain=air_density
  Gain2 : Gain  Gain=0.5
  Gain3 : Gain  Gain=S_seg3
  Math Function : Math  Operator=magnitude^2  SaturateOnIntegerOverflow=on
  p : Outport
  wires:
  Gain3/1 -> p/1
  Gain2/1 -> Gain3/1
  Gain1/1 -> Gain2/1
  Math Function/1 -> Gain1/1
  v/1 -> Math Function/1

== system TBS_SIM/Caipriha Airframe1/Aerodynamic Coefficient/Segment3L1/wing/wing ==
  Alpha : Inport
  Delta : Inport  Port=2
  airspeed : Inport  Port=3
  AirspeedLookup : PreLookup  BreakpointsData=as  BeginIndexSearchUsingPreviousIndexResult=on  ExtrapMethod=Linear
  AlphaLookup : PreLookup  BreakpointsData=alpha_vec_0  BeginIndexSearchUsingPreviousIndexResult=on  ExtrapMethod=Linear
  CD : Interpolation_n-D  NumberOfTableDimensions=3  Table=ORIGIN_CD  ExtrapMethod=Clip  DiagnosticForOutOfRangeInput=Warning  InternalRulePriority=Speed
      settings: InputPortMap=u0,u1,u2,u3,u4,u5
  CD1 : Interpolation_n-D  NumberOfTableDimensions=3  Table=ORIGIN_CM  ExtrapMethod=Clip  DiagnosticForOutOfRangeInput=Warning  InternalRulePriority=Speed
      settings: InputPortMap=u0,u1,u2,u3,u4,u5
  CL : Interpolation_n-D  NumberOfTableDimensions=3  Table=ORIGIN_CL  ExtrapMethod=Clip  DiagnosticForOutOfRangeInput=Warning  InternalRulePriority=Speed
      settings: InputPortMap=u0,u1,u2,u3,u4,u5
  DeltaLookup : PreLookup  BreakpointsData=ORIGIN_DELTA  BeginIndexSearchUsingPreviousIndexResult=on  ExtrapMethod=Linear
  cl : Outport
  cd : Outport  Port=2
  cm : Outport  Port=3
  wires:
  Alpha/1 -> AlphaLookup/1
  airspeed/1 -> AirspeedLookup/1
  DeltaLookup/1 -> CD1/5, CL/5, CD/5
  DeltaLookup/2 -> CD1/6, CL/6, CD/6
  CL/1 -> cl/1
  AirspeedLookup/1 -> CD1/1, CD/1, CL/1
  AirspeedLookup/2 -> CD1/2, CD/2, CL/2
  AlphaLookup/1 -> CD/3, CD1/3, CL/3
  AlphaLookup/2 -> CD1/4, CD/4, CL/4
  CD/1 -> cd/1
  CD1/1 -> cm/1
  Delta/1 -> DeltaLookup/1

== system TBS_SIM/Caipriha Airframe1/Aerodynamic Coefficient/Segment3R/right wing/DynamicPressure ==
  v : Inport
  Gain1 : Gain  Gain=air_density
  Gain2 : Gain  Gain=0.5
  Gain3 : Gain  Gain=S_seg3
  Math Function : Math  Operator=magnitude^2  SaturateOnIntegerOverflow=on
  p : Outport
  wires:
  Gain3/1 -> p/1
  Gain2/1 -> Gain3/1
  Gain1/1 -> Gain2/1
  Math Function/1 -> Gain1/1
  v/1 -> Math Function/1

== system TBS_SIM/Caipriha Airframe1/Aerodynamic Coefficient/Segment3R/right wing/wing ==
  Alpha : Inport
  Delta : Inport  Port=2
  airspeed : Inport  Port=3
  AirspeedLookup : PreLookup  BreakpointsData=as  BeginIndexSearchUsingPreviousIndexResult=on  ExtrapMethod=Linear
  AlphaLookup : PreLookup  BreakpointsData=alpha_vec_0  BeginIndexSearchUsingPreviousIndexResult=on  ExtrapMethod=Linear
  CD : Interpolation_n-D  NumberOfTableDimensions=3  Table=ORIGIN_CD  ExtrapMethod=Clip  DiagnosticForOutOfRangeInput=Warning  InternalRulePriority=Speed
      settings: InputPortMap=u0,u1,u2,u3,u4,u5
  CD1 : Interpolation_n-D  NumberOfTableDimensions=3  Table=ORIGIN_CM  ExtrapMethod=Clip  DiagnosticForOutOfRangeInput=Warning  InternalRulePriority=Speed
      settings: InputPortMap=u0,u1,u2,u3,u4,u5
  CL : Interpolation_n-D  NumberOfTableDimensions=3  Table=ORIGIN_CL  ExtrapMethod=Clip  DiagnosticForOutOfRangeInput=Warning  InternalRulePriority=Speed
      settings: InputPortMap=u0,u1,u2,u3,u4,u5
  DeltaLookup : PreLookup  BreakpointsData=ORIGIN_DELTA  BeginIndexSearchUsingPreviousIndexResult=on  ExtrapMethod=Linear
  cl : Outport
  cd : Outport  Port=2
  cm : Outport  Port=3
  wires:
  Alpha/1 -> AlphaLookup/1
  airspeed/1 -> AirspeedLookup/1
  DeltaLookup/1 -> CD1/5, CL/5, CD/5
  DeltaLookup/2 -> CD1/6, CL/6, CD/6
  CL/1 -> cl/1
  AirspeedLookup/1 -> CD1/1, CD/1, CL/1
  AirspeedLookup/2 -> CD1/2, CD/2, CL/2
  AlphaLookup/1 -> CD/3, CD1/3, CL/3
  AlphaLookup/2 -> CD1/4, CD/4, CL/4
  CD/1 -> cd/1
  CD1/1 -> cm/1
  Delta/1 -> DeltaLookup/1

== system TBS_SIM/Variant Control System/Transition/Trans/Cruise Controller/Cruise ==
  Ve : Inport
  Xe : Inport  Port=2
  DCM : Inport  Port=3
  pqr : Inport  Port=4
  V_b : Inport  Port=5
  Euler : Inport  Port=6
  Angle Conversion : aerolibconvert2/Angle Conversion  IU=rad  OU=deg
  Demux : Demux
  Demux2 : Demux  Outputs=3
  Mux1 : Mux  Inputs=2
  Mux3 : Mux  Inputs=2
  Saturation : Saturate  UpperLimit=10000  LowerLimit=0
  Saturation1 : Saturate  UpperLimit=10000  LowerLimit=0
  Saturation2 : Saturate  UpperLimit=16.5  LowerLimit=-23
  Saturation3 : Saturate  UpperLimit=16.5  LowerLimit=-23
  Terminator : Terminator
  map : MATLAB Function  TreatAsAtomicUnit=on
  nav : MATLAB Function  TreatAsAtomicUnit=on
  ve : Scope  NumInputPorts=3
  RS : Outport
  "Actuator " : Outport  Port=2
  wires:
  V_b/1 -> nav/3(v)
  map/1(output) -> Demux/1
  Saturation/1 -> Mux1/1
  Demux/1 -> Saturation/1
  Demux/2 -> Saturation1/1
  Saturation1/1 -> Mux1/2
  Saturation2/1 -> Mux3/1
  Demux/4 -> Saturation3/1
  Saturation3/1 -> Mux3/2
  Demux/3 -> Saturation2/1
  nav/1(output) -> map/1(F_des)
  Angle Conversion/1 -> nav/2(PRY)
  Demux2/1 -> ve/1
  Demux2/2 -> ve/2
  Demux2/3 -> ve/3
  Ve/1 -> Demux2/1
  Xe/1 -> nav/1(p)
  pqr/1 -> nav/4(pqr)
  Mux1/1 -> RS/1
  Mux3/1 -> "Actuator "/1
  Euler/1 -> Angle Conversion/1
  DCM/1 -> Terminator/1

== system TBS_SIM/Variant Control System/Transition/Trans/Transition Controller/Hover ==
  Ve : Inport
  Xe : Inport  Port=2
  DCM : Inport  Port=3
  pqr : Inport  Port=4
  des_v : Inport  Port=5
  des_p : Inport  Port=6
  Attitude controller : Subsystem
  Constant1 : Constant  Value=[0,0,0]
  Demux4 : Demux
  Direction Cosine Matrix to Rotation Angles : aerolibtransform2/Direction Cosine Matrix to Rotation Angles  rotationOrder=YZX  lim=Default
      settings: AttributesFormatString=Rotation Order: %<rotationOrder>
  Mux2 : Mux  Inputs=2
  Mux4 : Mux  Inputs=2
  Nav_controller(quad_axes) : Subsystem
  Ramp1 : simulink/Sources/Ramp  slope=18  start=0  X0=0
  Saturation1 : Saturate  UpperLimit=80
  Saturation4 : Saturate  UpperLimit=10000  LowerLimit=0
  Saturation5 : Saturate  UpperLimit=10000  LowerLimit=0
  Saturation6 : Saturate  UpperLimit=16.5  LowerLimit=-23
  Saturation7 : Saturate  UpperLimit=16.5  LowerLimit=-23
  Scope : Scope  NumInputPorts=2
  Sum : Sum  Inputs=-+|
  map1 : Subsystem
  RS : Outport
  "Actuator " : Outport  Port=2
  wires:
  Saturation6/1 -> Mux4/1
  map1/1(Act) -> Demux4/1
  Mux4/1 -> "Actuator "/1
  Saturation4/1 -> Mux2/1
  Ve/1 -> Nav_controller(quad_axes)/1(True velocity)
  Demux4/2 -> Saturation5/1
  Demux4/4 -> Saturation7/1
  Saturation7/1 -> Mux4/2
  Xe/1 -> Nav_controller(quad_axes)/2(True Position)
  Demux4/1 -> Saturation4/1
  Saturation5/1 -> Mux2/2
  DCM/1 -> Direction Cosine Matrix to Rotation Angles/1
  Nav_controller(quad_axes)/1(phi_des) -> Attitude controller/1(phi_des)
  Attitude controller/2("M_C ") -> map1/2(M_c)
  Demux4/3 -> Saturation6/1
  pqr/1 -> Attitude controller/5(pqr)
  Direction Cosine Matrix to Rotation Angles/1 -> Nav_controller(quad_axes)/5(True PRY), Attitude controller/4(PRY)
  Attitude controller/1(F_c) -> map1/1(F_c)
  Constant1/1 -> Attitude controller/6(des_pqr)
  Nav_controller(quad_axes)/3(F_des) -> Attitude controller/3(F_des)
  Mux2/1 -> RS/1
  des_v/1 -> Nav_controller(quad_axes)/3(Desired velocity)
  des_p/1 -> Nav_controller(quad_axes)/4(Desired Position)
  Saturation1/1 -> Sum/1
  Ramp1/1 -> Saturation1/1
  Nav_controller(quad_axes)/2("theta_des ") -> Scope/2, Sum/2  "before slope"
  Sum/1 -> Scope/1, Attitude controller/2(theta_des)  "Theta_des"

== system TBS_SIM/Variant Control System/Transition/Trans/Transition Controller/Hover/Attitude controller ==
  phi_des : Inport
  theta_des : Inport  Port=2
  F_des : Inport  Port=3
  PRY : Inport  Port=4
  pqr : Inport  Port=5
  des_pqr : Inport  Port=6
  Add : Sum  Inputs=+-
  Angle Conversion1 : aerolibconvert2/Angle Conversion  IU=rad  OU=deg
  Constant1 : Constant  Value=90
  Demux : Demux  Outputs=3
  Gain : Gain  Gain=[-0.05;0.07;0.08]
  Gain1 : Gain  Gain=[-0.4;-0.8;1.4]
  Gain2 : Gain  Gain=[0 0 1; 0 1 0; 1 0 0]  Multiplication=Matrix(K*u)
  Gain3 : Gain  Gain=-1
  Gain4 : Gain  Gain=-1
  Mux : Mux  Inputs=3
  Scope1 : Scope
  Scope2 : Scope
  error_phi : Sum  Inputs=-+
  error_phi1 : Sum  Inputs=-+
  error_pqr : Sum  Inputs=-+
  error_pqr1 : Sum  Inputs=-+
  F_c : Outport
  "M_C " : Outport  Port=2
  wires:
  F_des/1 -> F_c/1
  des_pqr/1 -> error_pqr/1
  pqr/1 -> error_pqr/2
  phi_des/1 -> error_phi/1
  theta_des/1 -> error_phi1/1
  error_phi1/1 -> Mux/2
  Gain/1 -> Add/1
  Gain1/1 -> Scope2/1, Add/2
  PRY/1 -> Angle Conversion1/1
  error_phi/1 -> Mux/1
  Gain4/1 -> Mux/3
  Mux/1 -> Scope1/1, Gain/1
  error_pqr/1 -> Gain2/1
  Gain2/1 -> Gain1/1
  Add/1 -> "M_C "/1
  Demux/2 -> Gain3/1
  Gain3/1 -> error_phi/2
  Demux/1 -> error_pqr1/2
  Constant1/1 -> error_pqr1/1
  error_pqr1/1 -> error_phi1/2
  Angle Conversion1/1 -> Demux/1
  Demux/3 -> Gain4/1

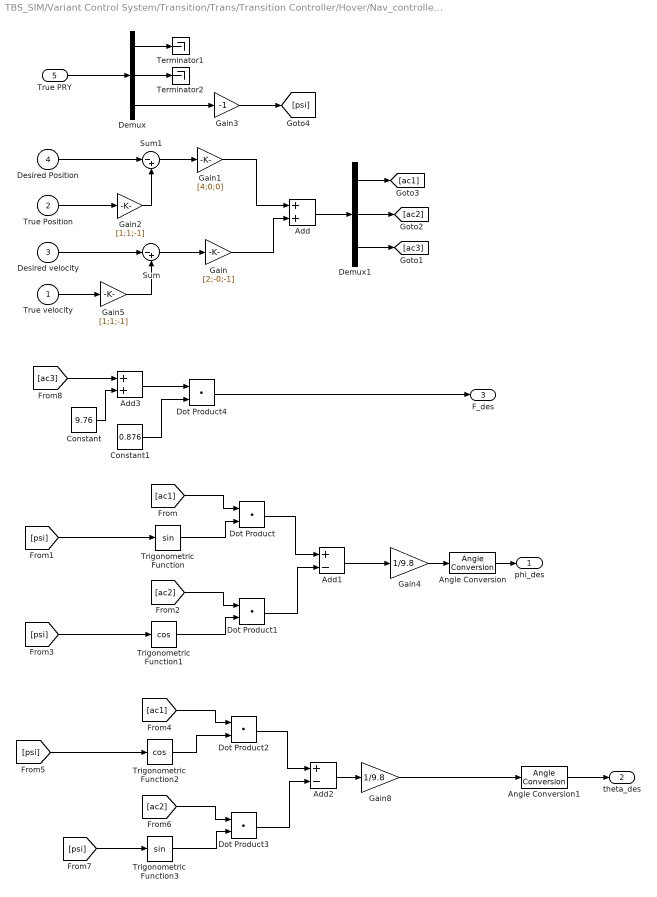
== system TBS_SIM/Variant Control System/Transition/Trans/Transition Controller/Hover/Nav_controller(quad_axes) ==
  True velocity : Inport
  True Position : Inport  Port=2
  Desired velocity : Inport  Port=3
  Desired Position : Inport  Port=4
  True PRY : Inport  Port=5
  Add : Sum
  Add1 : Sum  Inputs=+-
  Add2 : Sum  Inputs=+-
  Add3 : Sum
  Angle Conversion : aerolibconvert2/Angle Conversion  IU=rad  OU=deg
  Angle Conversion1 : aerolibconvert2/Angle Conversion  IU=rad  OU=deg
  Constant : Constant  Value=9.76
  Constant1 : Constant  Value=0.876
  Demux : Demux  Outputs=3
  Demux1 : Demux  Outputs=3
  Dot Product{,1..4} (5 alike) : DotProduct  InputSameDT=on  OutDataTypeStr=Inherit: Inherit via internal rule
  Gain : Gain  Gain=[2;-0;-1]
  Gain1 : Gain  Gain=[4;0;0]
  Gain2 : Gain  Gain=[1;1;-1]
  Gain3 : Gain  Gain=-1
  Gain4 : Gain  Gain=1/9.8
  Gain5 : Gain  Gain=[1;1;-1]
  Gain8 : Gain  Gain=1/9.8
  Sum : Sum  Inputs=|-+
  Sum1 : Sum  Inputs=|-+
  Terminator1 : Terminator
  Terminator2 : Terminator
  Trigonometric Function : Trigonometry
  Trigonometric Function1 : Trigonometry  Operator=cos
  Trigonometric Function2 : Trigonometry  Operator=cos
  Trigonometric Function3 : Trigonometry
  phi_des : Outport
  "theta_des " : Outport  Port=2
  F_des : Outport  Port=3
  wires:
  True velocity/1 -> Gain5/1
  Desired velocity/1 -> Sum/1
  Sum/1 -> Gain/1
  Sum1/1 -> Gain1/1
  Gain1/1 -> Add/1
  Gain/1 -> Add/2
  True PRY/1 -> Demux/1
  Demux/1 -> Terminator1/1
  Demux/3 -> Gain3/1
  Demux/2 -> Terminator2/1
  Add/1 -> Demux1/1
  Demux1/2 -> [ac2]
  [ac1] -> Dot Product/1
  Trigonometric Function/1 -> Dot Product/2
  [psi] -> Trigonometric Function/1
  [ac2] -> Dot Product1/1
  Trigonometric Function1/1 -> Dot Product1/2
  [psi] -> Trigonometric Function1/1
  Dot Product/1 -> Add1/1
  Dot Product1/1 -> Add1/2
  Add1/1 -> Gain4/1
  [ac1] -> Dot Product2/1
  Trigonometric Function2/1 -> Dot Product2/2
  [psi] -> Trigonometric Function2/1
  [ac2] -> Dot Product3/1
  Trigonometric Function3/1 -> Dot Product3/2
  [psi] -> Trigonometric Function3/1
  Dot Product2/1 -> Add2/1
  Dot Product3/1 -> Add2/2
  Add2/1 -> Gain8/1
  [ac3] -> Add3/1
  Constant/1 -> Add3/2
  Add3/1 -> Dot Product4/1
  Constant1/1 -> Dot Product4/2
  Dot Product4/1 -> F_des/1
  Demux1/1 -> [ac1]
  Demux1/3 -> [ac3]
  True Position/1 -> Gain2/1
  Gain2/1 -> Sum1/2
  Desired Position/1 -> Sum1/1
  Gain3/1 -> [psi]
  Gain4/1 -> Angle Conversion/1
  Angle Conversion/1 -> phi_des/1
  Gain8/1 -> Angle Conversion1/1
  Angle Conversion1/1 -> "theta_des "/1
  Gain5/1 -> Sum/2

== system TBS_SIM/Variant Control System/Transition/Trans/Transition Controller/Hover/map1 ==
  F_c : Inport
  M_c : Inport  Port=2
  Constant : Constant  Value=100
  Constant1 : Constant  Value=9.5
  Constant2 : Constant  Value=0.3
  Demux : Demux  Outputs=3
  Gain : Gain  Gain=1000
  Gain1 : Gain  Gain=1000
  Gain2 : Gain  Gain=50
  Gain3 : Gain  Gain=50
  Mux : Mux
  Sum : Sum  Inputs=-+|
  Sum1 : Sum  Inputs=|++
  Sum2 : Sum  Inputs=|+-
  Sum3 : Sum  Inputs=-+|
  Sum4 : Sum  Inputs=|++
  Sum5 : Sum  Inputs=|++
  Sum6 : Sum  Inputs=+-|
  Act : Outport
  wires:
  M_c/1 -> Demux/1
  F_c/1 -> Gain/1
  Demux/1 -> Gain1/1
  Gain1/1 -> Sum/2
  Constant/1 -> Sum/1
  Gain/1 -> Sum2/1, Sum1/1
  Sum/1 -> Sum1/2, Sum2/2
  Sum1/1 -> Mux/1
  Sum2/1 -> Mux/2
  Demux/2 -> Gain2/1
  Demux/3 -> Gain3/1
  Gain3/1 -> Sum4/1
  Constant1/1 -> Sum3/1
  Gain2/1 -> Sum3/2
  Constant2/1 -> Sum4/2
  Mux/1 -> Act/1
  Sum3/1 -> Sum5/1
  Sum4/1 -> Sum6/2, Sum5/2
  Sum5/1 -> Mux/4, Sum6/1
  Sum6/1 -> Mux/3

== matlab function TBS_SIM/Variant Control System/Cruise/Cruise/map ==
  data: F_des input; output output
function output  = ac(F_des)
%UNTITLED Summary of this function goes here
%   Detailed explanation goes here
% error_v=des_s(4:6)-s(4:6);
% k_v=[4 0 0;
%     5 0 0;
%     5 0 0];
% F_c=k_v(:,1).*error_v;
rs_mean=F_des(1)*2000;
deltars=F_des(4)*1000-100;
RS1=rs_mean+deltars;
RS2=rs_mean-deltars;
e=F_des(3)*50;
a=F_des(2)*50+0.3;
r=e-a;
l=e+a;
output=[RS1,RS2,r,l];
end

== matlab function TBS_SIM/Variant Control System/Cruise/Cruise/nav ==
  data: p input; PRY input; v input; output output; pqr input
function output   = slx_nav_controller( p,PRY,v,pqr)
%UNTITLED Summary of this function goes here
%   Detailed explanation goes here
height=-p(3);
eh=50-height;
ev=9-v(1);
des_t=4+0*eh+1*ev;
%des_t=2.8;
e_att=[0;8;0]-PRY;
des_M=zeros(3,1);
des_M(1)=0.08*e_att(1)-0.05*pqr(1);
des_M(2)=-0.1*e_att(2)+0.8*pqr(2);
des_M(3)=-0.1*e_att(3)+0.5*pqr(3);
output=[des_t;des_M];
end

== stateflow chart TBS_SIM/Variant Control System/Transition/Trans/Chart ==
  settings: executeAtInitialization=1
  state Transition
    during:
    trans_mode=1;
  state Cruise
    during:
    trans_mode=0;
  (default) -> Transition
  Transition -> Cruise : [v>2.5&&pitch<=30]
  data: v input; trans_mode output; pitch input

== matlab function TBS_SIM/Variant Control System/Transition/Trans/Cruise Controller/Cruise/map ==
  data: F_des input; output output
function output  = ac(F_des)
%UNTITLED Summary of this function goes here
%   Detailed explanation goes here
% error_v=des_s(4:6)-s(4:6);
% k_v=[4 0 0;
%     5 0 0;
%     5 0 0];
% F_c=k_v(:,1).*error_v;
rs_mean=F_des(1)*2000;
deltars=F_des(4)*1000-100;
RS1=rs_mean+deltars;
RS2=rs_mean-deltars;
e=F_des(3)*50;
a=F_des(2)*50+0.3;
r=e-a;
l=e+a;
output=[RS1,RS2,r,l];
end

== matlab function TBS_SIM/Variant Control System/Transition/Trans/Cruise Controller/Cruise/nav ==
  data: p input; PRY input; v input; output output; pqr input
function output   = slx_nav_controller( p,PRY,v,pqr)
%UNTITLED Summary of this function goes here
%   Detailed explanation goes here
height=-p(3);
eh=50-height;
ev=9-v(1);
des_t=4+0*eh+1*ev;
%des_t=2.8;
e_att=[0;8;0]-PRY;
des_M=zeros(3,1);
des_M(1)=0.08*e_att(1)-0.05*pqr(1);
des_M(2)=-0.1*e_att(2)+0.8*pqr(2);
des_M(3)=-0.1*e_att(3)+0.5*pqr(3);
output=[des_t;des_M];
end
